simulink model "sampleModel2066"  (R2023a)
settings: Solver=VariableStepAuto  StartTime=0.0  StopTime=10.0  RelTol=1e-3
libraries: hdlsllib x5, simulink x1
settings Model: Creator=user1  LastModifiedBy=user1

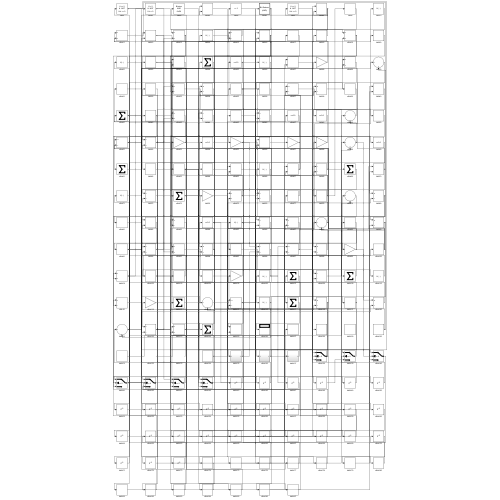
[thumbnail: Simulink's stored preview of the top-level diagram]
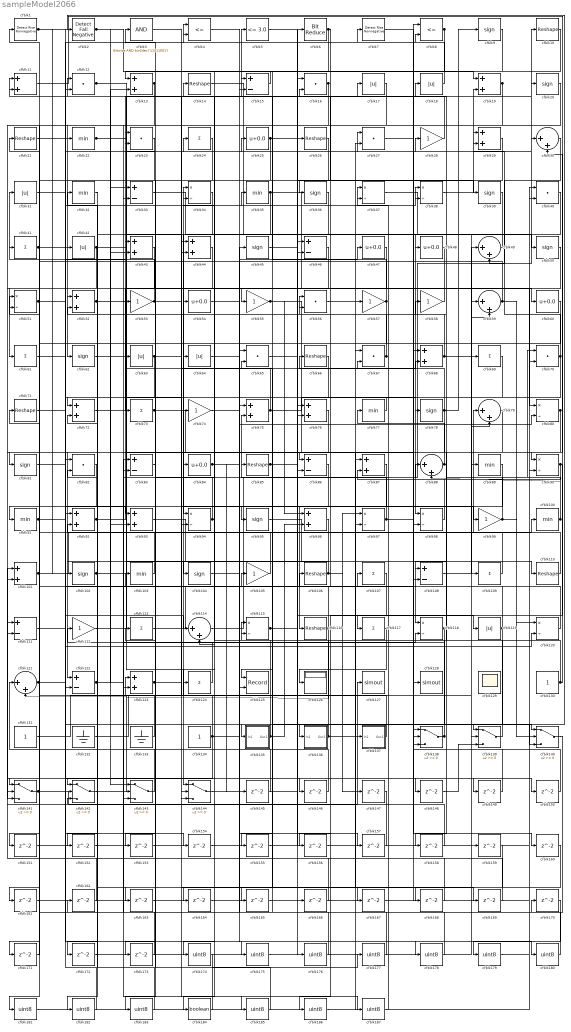
== system sampleModel2066 ==
  cfblk1 : hdlsllib/Logic and Bit Operations/Detect Rise Nonnegative  vinit=0  OutDataTypeStr=boolean
  cfblk{10,14,21,26,66,71,85,106,110,116} (10 alike) : Reshape
  cfblk{22,32,35,77,89,91,100,103} (8 alike) : MinMax
  cfblk{11,13,19,29,43..44,52,68,72,75..76,87,92..93,96,101,123} (17 alike) : Sum
  cfblk{9,20,36,39,45,50,62,78,81,95,102,104} (12 alike) : Signum
  cfblk{28,53,55,57..58,74,99,105,112} (9 alike) : Gain
  cfblk{24,41,61,69,73,107,109,113,117,124} (10 alike) : Sum  Inputs=+
  cfblk{15,33,46,83,86,108,111,122} (8 alike) : Sum  Inputs=+-
  cfblk{30,49,59,79,88,114,121} (7 alike) : Sum  Inputs=|++
  cfblk{34,37..38,51,80,90,94,97..98,115,118,120} (12 alike) : Product  Inputs=*/  RndMeth=Zero  SaturateOnIntegerOverflow=on
  cfblk{17..18,31,42,63..64,119} (7 alike) : Abs  SaturateOnIntegerOverflow=off
  cfblk{12,16,23,27,40,56,65,67,70,82} (10 alike) : DotProduct  OutDataTypeStr=Inherit: Inherit via internal rule
  cfblk125 : Record  FileSettingsInternal="{\"entries\":[{\"content\":{\"excelSettings\":{\"content\":{},\"type\":\"Streamout.ExcelSettings\"}},\"type\":\"Streamout.FileSettingStorage\",\"uuid\":\"\"}],\"packageUris\":[\"http:\\/\\/schema.mathworks.com\\/mf0\\/streamout_blocks\\/R2020a\"],\"version\":\"1.0\"}"  Layout=[1 1]  SignalsInternal="{\"entries\":[{\"content\":{\"signals\":[{\"content\":{\"blockPath\":[],\"dimensions\":[1],\"domain\":\"\",\"lineColor\":\"#a2142f\",\"plots\":[1],\"port\":1,\"signalID\":6450,\"signalName\":\"XY Graph:1\"},\"type\":\"RecordBlkView.Signal\",\"uuid\":\"\"},{\"content\":{\"blockPath\":[],\"dimensions\":[1],\"domain\":\"\",\"lineColor\":\"#139fff\",\"plots\":[1],\"port\":2,\"signalID\":6453,\"signalName\":\"XY Graph:2\"},\"type\":\"RecordBlkView.Signal\",\"uuid\":\"\"}]},\"type\":\"RecordBlkView.InputSignals\",\"uuid\":\"\"}],\"packageUris\":[\"http:\\/\\/schema.mathworks.com\\/mf0\\/streamout_blocks\\/R2020a\"],\"version\":\"1.0\"}"  VisualizationBindings="{\"xyplotplugin\":{\"info\":[{\"series\":[{\"bindingParametersList\":[{\"parameter\":\"X-Axis\",\"signalID\":6450,\"signalName\":\"XY Graph:1\"},{\"parameter\":\"Y-Axis\",\"signalID\":6453,\"signalName\":\"XY Graph:2\"}],\"seriesID\":9411}],\"subplotID\":1}]}}"  CompatibilityTag=XY  st=-1
  cfblk126 : Display
  cfblk127 : ToWorkspace  VariableName=simout  SaveFormat=Timeseries  SampleTime=-1
  cfblk128 : ToWorkspace  VariableName=simout  SaveFormat=Timeseries  SampleTime=-1
  cfblk129 : Scope
      settings: Floating=on
  cfblk130 : Constant  SampleTime=-1
  cfblk131 : Constant  SampleTime=-1
  cfblk132 : Ground
  cfblk133 : Ground
  cfblk134 : Constant  SampleTime=-1
  cfblk135 : Subsystem
      settings: LibrarySourceBlock=|
      | hdlsllib/Ports &
      | Subsystems/Subsystem
  cfblk136 : Subsystem
      settings: LibrarySourceBlock=|
      | hdlsllib/Ports &
      | Subsystems/Subsystem
  cfblk137 : Subsystem
      settings: LibrarySourceBlock=|
      | hdlsllib/Ports &
      | Subsystems/Subsystem
  cfblk{138..144} (7 alike) : Switch  SaturateOnIntegerOverflow=off  InputSameDT=off
  cfblk{145..173} (29 alike) : Delay  SampleTime=1
  cfblk{174..183,185..187} (13 alike) : DataTypeConversion  OutDataTypeStr=uint8  SaturateOnIntegerOverflow=off  RndMeth=Floor
  cfblk184 : DataTypeConversion  OutDataTypeStr=boolean  SaturateOnIntegerOverflow=off  RndMeth=Floor
  cfblk2 : hdlsllib/Logic and Bit Operations/Detect Fall Negative  vinit=0  OutDataTypeStr=boolean
  cfblk{25,47..48,54,60,84} (6 alike) : Bias  Bias=0.0  SaturateOnIntegerOverflow=off
  cfblk3 : simulink/Logic and Bit Operations/Bitwise Operator  logicop=AND  UseBitMask=on  BitMask=bin2dec('11011001')  BitMaskRealWorld=Stored Integer
      settings: LibrarySourceBlock=|
      | hdlsllib/Logic and Bit
      | Operations/Bitwise
      | Operator
  cfblk4 : RelationalOperator  Operator=<=  OutDataTypeStr=boolean  InputSameDT=off
  cfblk5 : hdlsllib/Logic and Bit Operations/Compare To Constant  relop=<=  const=3.0  OutDataTypeStr=boolean
  cfblk6 : hdlsllib/Logic and Bit Operations/Bit Reduce  mode=AND
  cfblk7 : hdlsllib/Logic and Bit Operations/Detect Rise Nonnegative  vinit=0  OutDataTypeStr=boolean
  cfblk8 : RelationalOperator  Operator=<=  OutDataTypeStr=boolean  InputSameDT=off
  wires:
  cfblk133/1 -> cfblk71/1
  cfblk63/1 -> cfblk68/2, cfblk122/2, cfblk99/1, cfblk167/1
  cfblk24/1 -> cfblk144/1
  cfblk92/1 -> cfblk17/1, cfblk33/1
  cfblk68/1 -> cfblk69/1, cfblk52/2
  cfblk76/1 -> cfblk122/1
  cfblk84/1 -> cfblk47/1, cfblk34/2, cfblk145/1
  cfblk141/1 -> cfblk127/1, cfblk24/1, cfblk120/2
  cfblk114/1 -> cfblk10/1
  cfblk11/1 -> cfblk90/1
  cfblk136/1(Out1) -> cfblk115/1, cfblk168/1
  cfblk41/1 -> cfblk42/1, cfblk175/1
  cfblk131/1 -> cfblk57/1
  cfblk87/1 -> cfblk116/1
  cfblk101/1 -> cfblk79/1, cfblk2/1
  cfblk40/1 -> cfblk98/1
  cfblk100/1 -> cfblk70/1, cfblk53/1, cfblk88/2
  cfblk72/1 -> cfblk86/1
  cfblk42/1 -> cfblk27/1, cfblk161/1
  cfblk121/1 -> cfblk106/1, cfblk35/1
  cfblk60/1 -> cfblk102/1
  cfblk134/1 -> cfblk34/1, cfblk141/3, cfblk80/2
  cfblk85/1 -> cfblk169/1, cfblk180/1
  cfblk15/1 -> cfblk13/1
  cfblk57/1 -> cfblk141/1, cfblk15/1
  cfblk39/1 -> cfblk94/1
  cfblk43/1 -> cfblk62/1
  cfblk112/1 -> cfblk30/1
  cfblk34/1 -> cfblk72/1
  cfblk115/1 -> cfblk6/1, cfblk119/1
  cfblk99/1 -> cfblk54/1, cfblk140/2, cfblk14/1
  cfblk137/1(Out1) -> cfblk123/1
  cfblk22/1 -> cfblk110/1, cfblk94/2
  cfblk62/1 -> cfblk5/1
  cfblk33/1 -> cfblk50/1
  cfblk8/1 -> cfblk7/1, cfblk76/2, cfblk4/2
  cfblk67/1 -> cfblk37/1, cfblk23/2
  cfblk13/1 -> cfblk143/3, cfblk151/1
  cfblk48/1 -> cfblk61/1
  cfblk46/1 -> cfblk73/1
  cfblk25/1 -> cfblk26/1, cfblk173/1
  cfblk106/1 -> cfblk104/1, cfblk97/1, cfblk147/1
  cfblk102/1 -> cfblk100/1, cfblk138/2
  cfblk52/1 -> cfblk144/3, cfblk43/2, cfblk187/1
  cfblk109/1 -> cfblk84/1
  cfblk49/1 -> cfblk48/1
  cfblk70/1 -> cfblk142/1, cfblk29/2
  cfblk53/1 -> cfblk31/1, cfblk38/2
  cfblk90/1 -> cfblk117/1, cfblk87/2
  cfblk88/1 -> cfblk77/1, cfblk158/1
  cfblk73/1 -> cfblk137/1(In1), cfblk140/3
  cfblk47/1 -> cfblk101/2
  cfblk95/1 -> cfblk118/1
  cfblk1/1 -> cfblk139/1, cfblk143/2
  cfblk118/1 -> cfblk115/2, cfblk156/1
  cfblk59/1 -> cfblk21/1, cfblk120/1
  cfblk64/1 -> cfblk45/1
  cfblk93/1 -> cfblk128/1
  cfblk139/1 -> cfblk103/1
  cfblk132/1 -> cfblk44/1
  cfblk20/1 -> cfblk52/1
  cfblk61/1 -> cfblk22/1
  cfblk75/1 -> cfblk78/1, cfblk23/1
  cfblk142/1 -> cfblk59/2
  cfblk66/1 -> cfblk144/2
  cfblk105/1 -> cfblk51/1
  cfblk144/1 -> cfblk86/2
  cfblk12/1 -> cfblk60/1, cfblk143/1
  cfblk55/1 -> cfblk138/1, cfblk96/1
  cfblk94/1 -> cfblk63/1, cfblk184/1
  cfblk78/1 -> cfblk66/1, cfblk56/2, cfblk9/1, cfblk138/3
  cfblk56/1 -> cfblk38/1
  cfblk37/1 -> cfblk109/1
  cfblk120/1 -> cfblk16/2
  cfblk124/1 -> cfblk72/2
  cfblk17/1 -> cfblk44/2
  cfblk18/1 -> cfblk8/2
  cfblk36/1 -> cfblk125/1
  cfblk28/1 -> cfblk12/1
  cfblk44/1 -> cfblk83/2
  cfblk14/1 -> cfblk76/1
  cfblk143/1 -> cfblk32/1
  cfblk98/1 -> cfblk67/2
  cfblk2/1 -> cfblk19/1, cfblk93/2
  cfblk80/1 -> cfblk108/1, cfblk171/1
  cfblk69/1 -> cfblk108/2
  cfblk16/1 -> cfblk124/1, cfblk46/2, cfblk33/2
  cfblk58/1 -> cfblk55/1
  cfblk97/1 -> cfblk75/2, cfblk20/1
  cfblk119/1 -> cfblk51/2, cfblk155/1
  cfblk116/1 -> cfblk121/2, cfblk105/1
  cfblk38/1 -> cfblk19/2
  cfblk19/1 -> cfblk141/2, cfblk164/1
  cfblk122/1 -> cfblk118/2, cfblk88/1, cfblk13/2, cfblk150/1
  cfblk21/1 -> cfblk135/1(In1)
  cfblk135/1(Out1) -> cfblk11/1, cfblk96/2
  cfblk117/1 -> cfblk126/1
  cfblk26/1 -> cfblk95/1
  cfblk77/1 -> cfblk74/1
  cfblk110/1 -> cfblk56/1
  cfblk108/1 -> cfblk89/1
  cfblk81/1 -> cfblk43/1
  cfblk10/1 -> cfblk64/1
  cfblk30/1 -> cfblk49/2
  cfblk113/1 -> cfblk68/1
  cfblk79/1 -> cfblk111/2
  cfblk103/1 -> cfblk92/2
  cfblk130/1 -> cfblk30/2, cfblk58/1
  cfblk54/1 -> cfblk136/1(In1)
  cfblk123/1 -> cfblk18/1, cfblk148/1
  cfblk86/1 -> cfblk125/2
  cfblk51/1 -> cfblk29/1, cfblk154/1
  cfblk138/1 -> cfblk112/1, cfblk85/1
  cfblk35/1 -> cfblk80/1, cfblk114/2, cfblk39/1
  cfblk89/1 -> cfblk91/1
  cfblk31/1 -> cfblk25/1
  cfblk71/1 -> cfblk28/1
  cfblk5/1 -> cfblk140/1
  cfblk111/1 -> cfblk12/2
  cfblk91/1 -> cfblk114/1, cfblk4/1, cfblk93/1
  cfblk6/1 -> cfblk36/1, cfblk15/2
  cfblk23/1 -> cfblk81/1
  cfblk145/1 -> cfblk92/1
  cfblk104/1 -> cfblk146/1
  cfblk146/1 -> cfblk121/1
  cfblk147/1 -> cfblk142/3
  cfblk148/1 -> cfblk139/3
  cfblk7/1 -> cfblk149/1
  cfblk149/1 -> cfblk8/1
  cfblk150/1 -> cfblk139/2
  cfblk151/1 -> cfblk123/2
  cfblk32/1 -> cfblk152/1
  cfblk152/1 -> cfblk16/1
  cfblk29/1 -> cfblk153/1
  cfblk153/1 -> cfblk59/1
  cfblk154/1 -> cfblk46/1
  cfblk155/1 -> cfblk90/2
  cfblk156/1 -> cfblk79/2
  cfblk74/1 -> cfblk157/1
  cfblk157/1 -> cfblk101/1
  cfblk158/1 -> cfblk142/2
  cfblk27/1 -> cfblk160/1
  cfblk161/1 -> cfblk97/2
  cfblk140/1 -> cfblk162/1
  cfblk162/1 -> cfblk111/1
  cfblk50/1 -> cfblk163/1
  cfblk163/1 -> cfblk87/1
  cfblk164/1 -> cfblk70/2
  cfblk9/1 -> cfblk165/1
  cfblk165/1 -> cfblk98/2
  cfblk45/1 -> cfblk166/1
  cfblk166/1 -> cfblk1/1
  cfblk167/1 -> cfblk49/1
  cfblk168/1 -> cfblk37/2
  cfblk169/1 -> cfblk75/1
  cfblk171/1 -> cfblk11/2
  cfblk96/1 -> cfblk172/1
  cfblk172/1 -> cfblk67/1
  cfblk173/1 -> cfblk83/1
  cfblk159/1 -> cfblk174/1
  cfblk175/1 -> cfblk159/1
  cfblk65/1 -> cfblk176/1
  cfblk176/1 -> cfblk41/1
  cfblk174/1 -> cfblk177/1
  cfblk177/1 -> cfblk65/1
  cfblk4/1 -> cfblk178/1
  cfblk178/1 -> cfblk65/2
  cfblk170/1 -> cfblk179/1
  cfblk179/1 -> cfblk40/2
  cfblk180/1 -> cfblk170/1
  cfblk82/1 -> cfblk181/1
  cfblk181/1 -> cfblk40/1
  cfblk160/1 -> cfblk182/1
  cfblk182/1 -> cfblk82/1
  cfblk83/1 -> cfblk183/1
  cfblk183/1 -> cfblk82/2
  cfblk184/1 -> cfblk3/1
  cfblk3/1 -> cfblk185/1
  cfblk185/1 -> cfblk113/1
  cfblk107/1 -> cfblk186/1
  cfblk186/1 -> cfblk27/2
  cfblk187/1 -> cfblk107/1

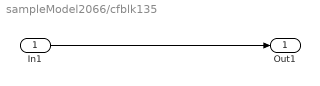
== system sampleModel2066/cfblk135 ==
  In1 : Inport
  Out1 : Outport
  wires:
  In1/1 -> Out1/1

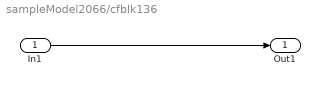
== system sampleModel2066/cfblk136 ==
  In1 : Inport
  Out1 : Outport
  wires:
  In1/1 -> Out1/1

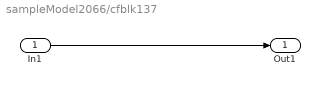
== system sampleModel2066/cfblk137 ==
  In1 : Inport
  Out1 : Outport
  wires:
  In1/1 -> Out1/1
